simulink model "xmenora0lubricado"  (R2022a)
settings: Solver=VariableStepAuto  StartTime=0.0  StopTime=5.0  RelTol=1e-3
settings Model: Creator=melaaa  LastModifiedBy=melaaa

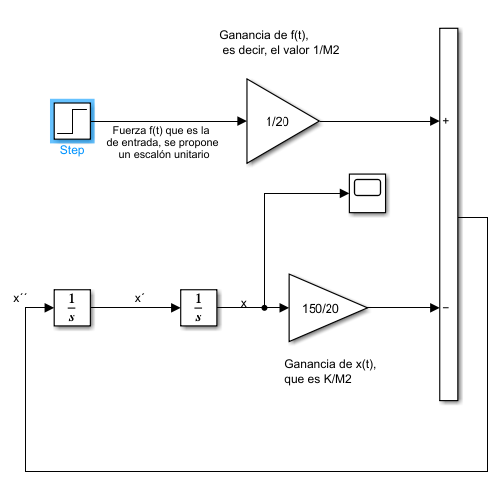
[thumbnail: Simulink's stored preview of the top-level diagram]
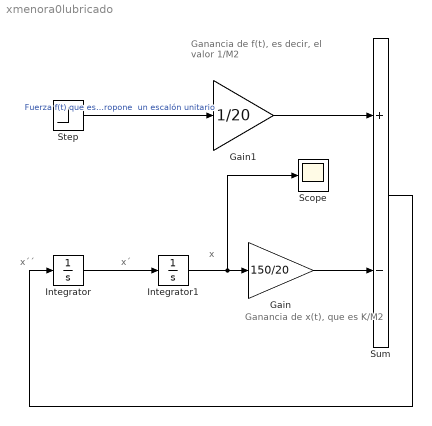
== system xmenora0lubricado ==
  note: Ganancia de x(t),
      | que es K/M2
  note: x
  note: x´
  note: x´´
  note: Ganancia de f(t),
      |  es decir, el valor 1/M2
  Gain : Gain  Gain=150/20
  Gain1 : Gain  Gain=1/20
  Integrator : Integrator
  Integrator1 : Integrator
  Scope : Scope
  Step : Step  Time=0  SampleTime=0
  Sum : Sum  Inputs=+-
  wires:
  Integrator/1 -> Integrator1/1
  Step/1 -> Gain1/1  "Fuerza f(t) que es la  de entrada, se propone  un escalón unitario"
  Gain1/1 -> Sum/1
  Sum/1 -> Integrator/1
  Integrator1/1 -> Scope/1, Gain/1
  Gain/1 -> Sum/2
